simulink model "BPSK_RC"  (R2014b)
settings: Solver=ode45  StartTime=0.0  StopTime=1  RelTol=1e-3
libraries: commdigbbndpm3 x2, commfilt2 x2, commchan3 x1, commsink2 x1, commrandsrc2 x1
settings Model: Creator=zinab rabie  LastModifiedBy=zinab rabie

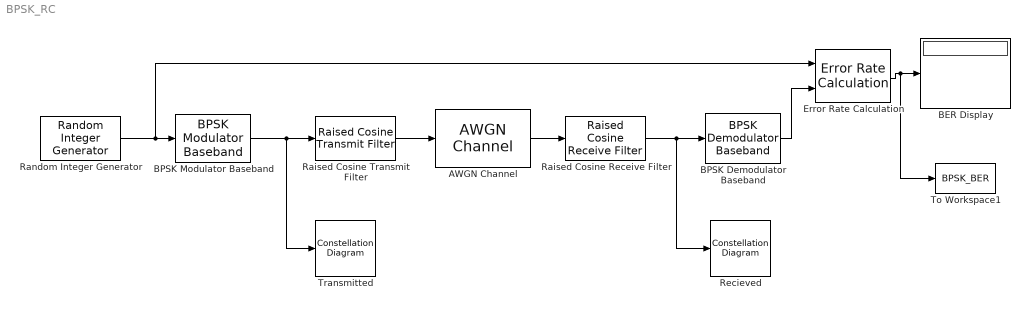
== system BPSK_RC ==
  AWGN Channel : commchan3/AWGN Channel  InputProcessing=Columns as channels (frame based)  seed=67  noiseMode="Signal to noise ratio  (Eb/No)"  EbNodB=EbNo  EsNodB=10  SNRdB=10  bitsPerSym=1  Ps=1  Tsym=1  variance=1
  BER Display : Display
  BPSK Demodulator Baseband : commdigbbndpm3/BPSK Demodulator Baseband  Ph=0  DecType=Hard decision  VarSource=Dialog  Variance=1  outDtype=Inherit via internal rule  derotateFactorWordLen=16
  BPSK Modulator Baseband : commdigbbndpm3/BPSK Modulator Baseband  Ph=0  outDtype=double  outWordLen=16  outUDDataType=sfix(16)  outFracLenMode=Best precision  outFracLen=15
  Error Rate Calculation : commsink2/Error Rate Calculation  N=16  st_delay=0  cp_mode=Entire frame  subframe=[]  PMode=Port  WsName=ErrorVec  RsMode2=off  stop=on  numErr=maxNumErrs  maxBits=maxNumBits
  Raised Cosine Receive Filter : commfilt2/Raised Cosine Receive Filter  filtType=Square root  N=2  filtSpan=16  currentFiltSpan=16  D=(16)/2  R=0.5  sampMode=Mute  saveAsFlag=0  rateMode=Downsampling  downFactor=2  downOffset=0  framing=Enforce single-rate processing  InputProcessing=Columns as channels (frame based)  checkGain=Normalized  filterGain=1  checkCoeff=off  variableName=rcRxFilt  launchFVT=on  roundingMode=Floor  overflowMode=off
  Raised Cosine Transmit Filter : commfilt2/Raised Cosine Transmit Filter  filtType=Square root  filtSpan=16  currentFiltSpan=16  D=(16)/2  R=0.5  sampMode=Mute  saveAsFlag=0  N=2  framing=Enforce single-rate processing  InputProcessing=Columns as channels (frame based)  checkGain=Normalized  filterGain=1  checkCoeff=off  variableName=rcTxFilt  launchFVT=on  roundingMode=Floor  overflowMode=off
  Random Integer Generator : commrandsrc2/Random Integer Generator  mul=2  seed=67  Ts=1  frameBased=on  sampPerFrame=1000  orient=off  outDataType=double
  Recieved : ConstellationDiagram
  To Workspace1 : ToWorkspace  VariableName=BPSK_BER  SampleTime=-1
      settings: Save2DSignal=2-D array (concatenate along first dimension)
  Transmitted : ConstellationDiagram
  wires:
  BPSK Modulator Baseband/1 -> Transmitted/1, Raised Cosine Transmit Filter/1
  BPSK Demodulator Baseband/1 -> Error Rate Calculation/2
  Error Rate Calculation/1 -> To Workspace1/1, BER Display/1
  Random Integer Generator/1 -> Error Rate Calculation/1, BPSK Modulator Baseband/1
  AWGN Channel/1 -> Raised Cosine Receive Filter/1
  Raised Cosine Transmit Filter/1 -> AWGN Channel/1
  Raised Cosine Receive Filter/1 -> Recieved/1, BPSK Demodulator Baseband/1
